simulink model "segway_complimentarry_filter"  (Simulink 8.1)
settings: Solver=ode45  StartTime=0.0  StopTime=inf  RelTol=1e-3
StartFcn:
  | %The GUI handles are by default hidden, turn them on
  | set(0,'ShowHiddenHandles','on');
  | 
  | %Set up the arguments that will go into the gain block event callback listener
  | blk = 'segway_complimentarry_filter/Out1';
  | event = 'PostOutputs';
  | listener = @updategui;
  | 
  | %Create the listener
  | h = add_exec_event_listener(blk, event, listener);
undefined symbols (not defined in the file or in its folder): eingang
settings Model: Creator=Emanuel  LastModifiedBy=Lauber
settings DebuggingCC: FcnCallInpInsideContextMsg=EnableAllAsWarning
settings RTWCC: GenerateReport=on  LaunchReport=on  TargetLang=C++  RTWCompilerOptimization=On
settings GRTTargetCC: CombineOutputUpdateFcns=on  GRTInterface=off

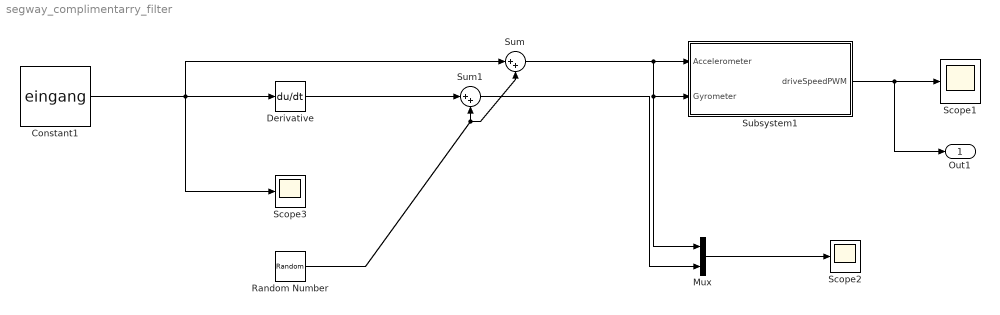
== system segway_complimentarry_filter ==
  Constant1 : Constant  Value=eingang  OutDataTypeStr=double
  Derivative : Derivative
  Mux : Mux  Inputs=2
  Random Number : RandomNumber  Variance=0  SampleTime=0.1
  Scope1 : Scope
      settings: YMin=0  YMax=35
  Scope2 : Scope
      settings: YMin=-0.5  YMax=0.05  SaveName=ScopeData2
  Scope3 : Scope
      settings: YMin=-0.105  YMax=-0.095
  Subsystem1 : Subsystem
  Sum : Sum  Inputs=|++
  Sum1 : Sum  Inputs=|++
  Out1 : Outport
  wires:
  Derivative/1 -> Sum1/1
  Mux/1 -> Scope2/1
  Random Number/1 -> Sum1/2, Sum/2
  Sum/1 -> Mux/1, Subsystem1/2(Gyrometer), Subsystem1/1(Accelerometer)
  Sum1/1 -> Mux/2
  Constant1/1 -> Scope3/1, Derivative/1, Sum/1
  Subsystem1/1(driveSpeedPWM) -> Out1/1, Scope1/1

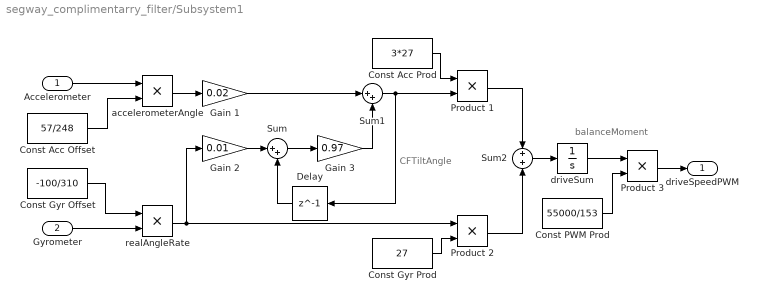
== system segway_complimentarry_filter/Subsystem1 ==
  note: balanceMoment
  note: CFTiltAngle
  Accelerometer : Inport
  Gyrometer : Inport  Port=2
  Const Acc Offset : Constant  Value=57/248
  Const Acc Prod : Constant  Value=3*27
  Const Gyr Offset : Constant  Value=-100/310
  Const Gyr Prod : Constant  Value=27
  Const PWM Prod : Constant  Value=55000/153
  Delay : Delay  DelayLength=1  InitialCondition=0  SampleTime=0.001
  Gain 1 : Gain  Gain=0.02
  Gain 2 : Gain  Gain=0.01
  Gain 3 : Gain  Gain=0.97
  Product 1 : Product
  Product 2 : Product
  Product 3 : Product
  Sum : Sum  Inputs=|++
  Sum1 : Sum  Inputs=|++
  Sum2 : Sum
  accelerometerAngle : Product
  driveSum : Integrator
  realAngleRate : Product
  driveSpeedPWM : Outport
  wires:
  Gyrometer/1 -> realAngleRate/2
  Const Gyr Offset/1 -> realAngleRate/1
  Const Acc Offset/1 -> accelerometerAngle/2
  Accelerometer/1 -> accelerometerAngle/1
  realAngleRate/1 -> Gain 2/1, Product 2/1
  Gain 2/1 -> Sum/1
  Sum/1 -> Gain 3/1
  accelerometerAngle/1 -> Gain 1/1
  Gain 1/1 -> Sum1/1
  Gain 3/1 -> Sum1/2
  Sum1/1 -> Delay/1, Product 1/2
  Delay/1 -> Sum/2
  Const Acc Prod/1 -> Product 1/1
  Const Gyr Prod/1 -> Product 2/2
  Product 1/1 -> Sum2/1
  Product 2/1 -> Sum2/2
  Sum2/1 -> driveSum/1
  driveSum/1 -> Product 3/1
  Const PWM Prod/1 -> Product 3/2
  Product 3/1 -> driveSpeedPWM/1
